simulink model "Bai_6"  (R2020b)
settings: Solver=VariableStepAuto  StartTime=0.0  StopTime=5  RelTol=1e-3
undefined symbols (not defined in the file): F, Ti
settings Model: Creator=John Andrew  LastModifiedBy=John Andrew

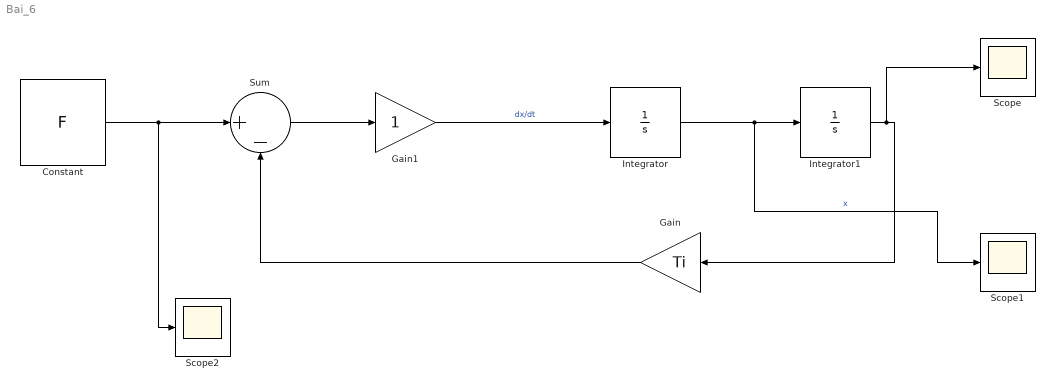
== system Bai_6 ==
  Constant : Constant  Value=F
  Gain : Gain  Gain=Ti
  Gain1 : Gain
  Integrator : Integrator
  Integrator1 : Integrator
  Scope : Scope
  Scope1 : Scope
  Scope2 : Scope
  Sum : Sum  Inputs=|+-
  wires:
  Constant/1 -> Scope2/1, Sum/1
  Integrator/1 -> Scope1/1, Integrator1/1  "x"
  Integrator1/1 -> Scope/1, Gain/1
  Gain/1 -> Sum/2
  Sum/1 -> Gain1/1
  Gain1/1 -> Integrator/1  "dx/dt"
